simulink model "working_kalman_old"  (R2025b)
settings: Solver=FixedStepDiscrete  StartTime=0.0  StopTime=+inf  FixedStep=simulink_Ts  RelTol=1e-3  EnableMultiTasking=on
InitFcn:
  | InitSensorFusion
values from neighbouring files (symbols this model uses):
  avg_order = 2    [InitSensorFusion_old.m]
  d = 0.15*sqrt(2)/2    [InitSensorFusion_old.m]
  friction_offset = 0.0001    [InitSensorFusion_old.m]
  friction_slope = 0.023e-3    (= 2.3e-05)    [InitSensorFusion_old.m]
  g = 9.81    [InitSensorFusion_old.m]
  Ic0 = Is0 + Iw0 - Iwg    [InitSensorFusion_old.m]
  ICM42_g = 9.8121    [InitSensorFusion_old.m]
  ICM42_gyr_offset = [-0.1319, -0.6878, 0.1737]    [InitSensorFusion_old.m]
  ICM42_params = params_1period    [InitSensorFusion_old.m]
  init_acc_bias = [0 0 0]'    [InitSensorFusion_old.m]
  init_P = P_initial    (= 10)    [InitSensorFusion_old.m]
  init_rot_quat = [0 0 0 1]'    [InitSensorFusion_old.m]
  kalman_Ts = 0.01    [InitSensorFusion_old.m]
  KV = 330    [InitSensorFusion_old.m]
  mc = mw + ms    (= 0.55)    [InitSensorFusion_old.m]
  sensor_Ts = 0.01    [InitSensorFusion_old.m]
  simulink_Ts = 0.01    [InitSensorFusion_old.m]
  stateInit = StateEnum.Initialization    [InitSensorFusion_old.m]
undefined symbols (not defined in the file or in its folder): init_time, StateEnum
libraries: mbedblockslib x24, stmnucleof7lib x5, nucleoutilitieslib x5, canmsglib x4, simulink x3, visionstatistics x2
(part 1 of 2)
settings Model: SimulationMode=external  ExtModeTrigDuration=10  Creator=dozav  LastModifiedBy=dozav
settings SolverCC: AutoInsertRateTranBlk=on
settings DataIOCC: SaveOutput=off  DSMLogging=off  ReturnWorkspaceOutputs=off  LoggingFileName=loggedData.mat
settings OptimizationCC: DefaultParameterBehavior=Inlined  EnhancedBackFolding=on  PassReuseOutputArgsAs=Individual arguments  ZeroExternalMemoryAtStartup=off  ZeroInternalMemoryAtStartup=off  MaxStackSize=64  OptimizeBlockOrder=speed  DifferentSizesBufferReuse=on  OptimizationCustomize=off  EfficientTunableParamExpr=on
settings DebuggingCC: ParameterTunabilityLossMsg=error
settings HardwareCC: ProdBitPerPointer=32.0  ProdBitPerSizeT=32.0  ProdBitPerPtrDiffT=32.0  ProdLargestAtomicInteger=Long  ProdLargestAtomicFloat=Double  ProdWordSize=32.0  ProdLongLongMode=on  ProdHWDeviceType=ARM Compatible->ARM Cortex-M
settings ModelReferenceCC: UpdateModelReferenceTargets=Force
settings SFSimCC: MATLABDynamicMemAlloc=off
settings RTWCC: SystemTargetFile=ert.tlc  HardwareBoard=STM32 Nucleo F767ZI  TemplateMakefile=ert_default_tmf  Toolchain=GNU Tools for ARM Embedded Processors  Description=Embedded Coder
settings CodeAppCC: ForceParamTrailComments=on  IgnoreCustomStorageClasses=off  OperatorAnnotations=on  SimulinkDataObjDesc=on  SFDataObjDesc=on  InsertBlockDesc=on
settings ERTTargetCC: ExtModeTransport=3.0  ExtModeStaticAlloc=on  ExtModeStaticAllocSize=2000.0  ExtModeMexFile=ext_xcp  ExtModeIntrfLevel=Level2 - Open  TargetLangStandard=C99 (ISO)

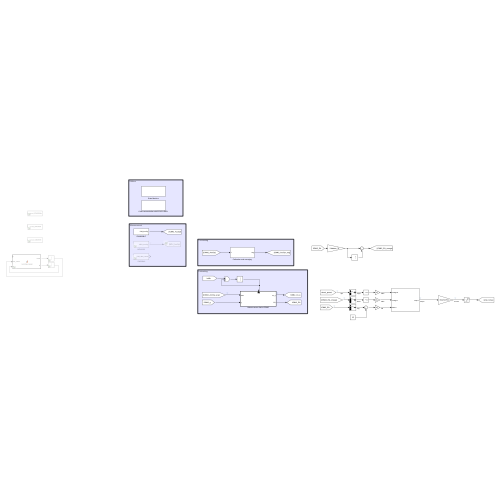
[thumbnail: Simulink's stored preview of the top-level diagram]
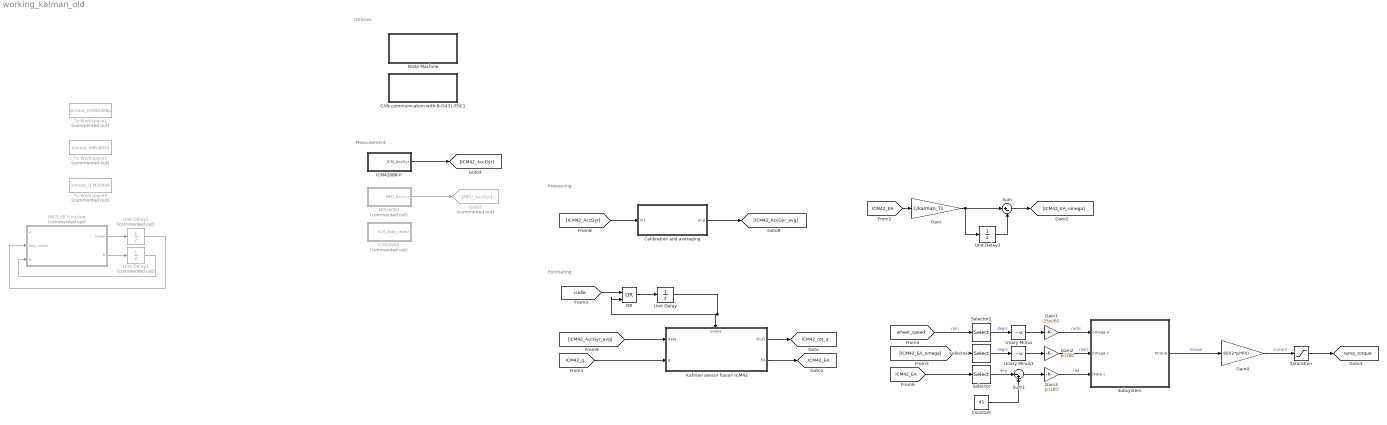
== system working_kalman_old ==
  note: Utilities
  note: Estimating
  note: Processing
  note: Measurement
  CAN communication with B-G431-ESC1 : Subsystem
  Calibration and averaging : Subsystem
  Constant : Constant  Value=45
  Gain : Gain  Gain=1/kalman_Ts
  Gain1 : Gain  Gain=2*pi/60
  Gain2 : Gain  Gain=pi/180
  Gain3 : Gain  Gain=pi/180
  Gain4 : Gain  Gain=60/(2*pi*KV)
  Goto5 : Goto  Commented=on  GotoTag=MPU_AccGyr
  ICM20948 : Subsystem  Commented=on
  ICM42688-P : Subsystem
  Kalman sensor fusion ICM42 : Subsystem
  MATLAB Function : MATLAB Function  Commented=on  TreatAsAtomicUnit=on
  MPU6050 : Subsystem  Commented=on
  OR : Logic  Operator=OR  IconShape=distinctive  AllPortsSameDT=off  OutDataTypeStr=boolean
  Saturation : Saturate  UpperLimit=1.5  LowerLimit=-1.5
  Selector : Selector  InputPortWidth=3  IndexOptions=Index vector (dialog)  Indices=[1]  OutputSizes=1
  Selector1 : Selector  InputPortWidth=3  IndexOptions=Index vector (dialog)  Indices=[1]  OutputSizes=1
  Selector2 : Selector  InputPortWidth=2  IndexOptions=Index vector (dialog)  Indices=[1]  OutputSizes=1
  State Machine : Subsystem
  Subsystem : Subsystem
  Sum : Sum  Inputs=|+-
  Sum1 : Sum  Inputs=|-+
  To Workspace1 : ToWorkspace  Commented=on  VariableName=simout_ICM42688p  SampleTime=-1
  To Workspace2 : ToWorkspace  Commented=on  VariableName=simout_MPU6050  SampleTime=-1
  To Workspace3 : ToWorkspace  Commented=on  VariableName=simout_ICM20948  SampleTime=-1
  Unary Minus : UnaryMinus
  Unary Minus1 : UnaryMinus
  Unit Delay : UnitDelay  SampleTime=-1  HasFrameUpgradeWarning=on
  Unit Delay1 : UnitDelay  Commented=on  SampleTime=-1  HasFrameUpgradeWarning=on
  Unit Delay2 : UnitDelay  Commented=on  SampleTime=-1  HasFrameUpgradeWarning=on
  Unit Delay3 : UnitDelay  InitialCondition=zeros(1,3)  SampleTime=kalman_Ts  HasFrameUpgradeWarning=on
  tag scope: ICM42_EA=global, ICM42_rot_q=global, ramp_torque=global
  wires:
  ICM42688-P/1(ICM_AccGyr) -> [ICM42_AccGyr]
  MATLAB Function/2(N) -> Unit Delay1/1
  MATLAB Function/1(mean) -> Unit Delay2/1
  Unit Delay1/1 -> MATLAB Function/3("N ")
  Unit Delay2/1 -> MATLAB Function/2(last_mean)
  [ICM42_g] -> Kalman sensor fusion ICM42/2(g)
  [ICM42_AccGyr_avg] -> Kalman sensor fusion ICM42/1(data)
  MPU6050/1(MPU_AccGyr) -> Goto5/1
  [isIdle] -> OR/1
  OR/1 -> Unit Delay/1
  Unit Delay/1 -> OR/2, Kalman sensor fusion ICM42/Enable
  [ICM42_AccGyr] -> Calibration and averaging/1(In1)
  Calibration and averaging/1(avg) -> [ICM42_AccGyr_avg]
  Kalman sensor fusion ICM42/1(Out1) -> [ICM42_rot_q]
  Kalman sensor fusion ICM42/2(EA) -> [ICM42_EA]
  [ICM42_EA] -> Gain/1
  Unit Delay3/1 -> Sum/2
  Sum/1 -> [ICM42_EA_omega]
  Gain/1 -> Sum/1, Unit Delay3/1
  [ICM42_EA] -> Selector/1
  [ICM42_EA_omega] -> Selector1/1
  [wheel_speed] -> Selector2/1  "rpm"
  Selector1/1 -> Unary Minus1/1  "deg/s"
  Gain1/1 -> Subsystem/1(omega w)  "rad/s"
  Gain2/1 -> Subsystem/2(omega c)  "rad/s"
  Gain3/1 -> Subsystem/3(theta c)  "rad"
  Selector2/1 -> Unary Minus/1  "deg/s"
  Subsystem/1(torque) -> Gain4/1  "torque"
  Gain4/1 -> Saturation/1  "current"
  Saturation/1 -> [ramp_torque]
  Unary Minus/1 -> Gain1/1
  Unary Minus1/1 -> Gain2/1
  Selector/1 -> Sum1/1  "deg"
  Sum1/1 -> Gain3/1
  Constant/1 -> Sum1/2

== system working_kalman_old/CAN communication with B-G431-ESC1 ==
  Receive CAN Messages : Subsystem
  Send CAN Messages : Subsystem

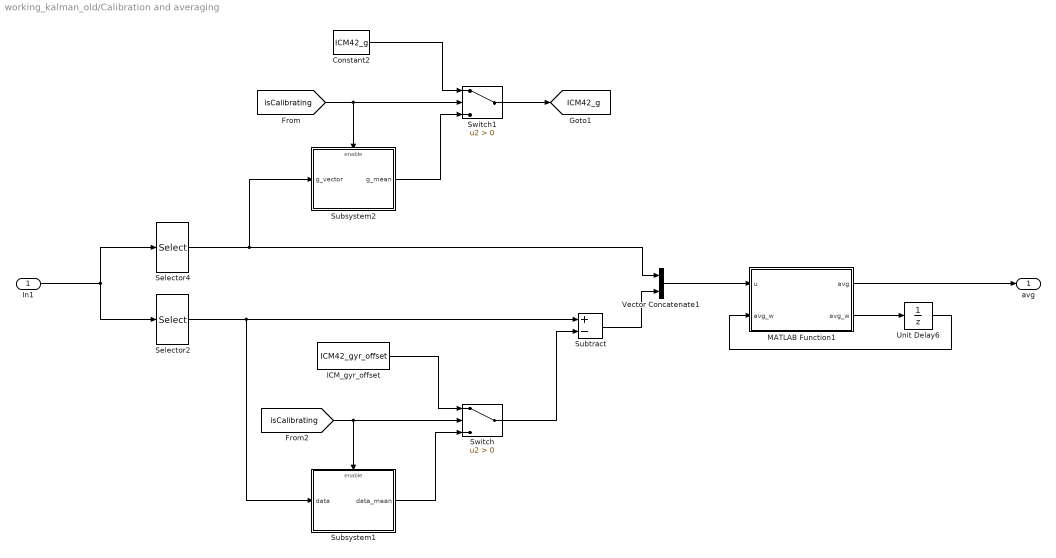
== system working_kalman_old/Calibration and averaging ==
  In1 : Inport
  Constant2 : Constant  Value=ICM42_g  SampleTime=-1
  ICM_gyr_offset : Constant  Value=ICM42_gyr_offset  SampleTime=-1
  MATLAB Function1 : MATLAB Function  TreatAsAtomicUnit=on
  Selector2 : Selector  InputPortWidth=6  IndexOptions=Starting index (dialog)  Indices=[4]  OutputSizes=3
  Selector4 : Selector  InputPortWidth=6  IndexOptions=Starting index (dialog)  Indices=[1]  OutputSizes=3
  Subsystem1 : Subsystem
  Subsystem2 : Subsystem
  Subtract : Sum  Inputs=+-
  Switch : Switch  Criteria=u2 > Threshold  SaturateOnIntegerOverflow=off  InputSameDT=off
  Switch1 : Switch  Criteria=u2 > Threshold  SaturateOnIntegerOverflow=off  InputSameDT=off
  Unit Delay6 : UnitDelay  InitialCondition=zeros(avg_order, 6)  SampleTime=-1  HasFrameUpgradeWarning=on
  Vector Concatenate1 : Concatenate
  avg : Outport
  tag scope: ICM42_g=global
  wires:
  Switch/1 -> Subtract/2
  MATLAB Function1/1(avg) -> avg/1
  Constant2/1 -> Switch1/1
  Subsystem1/1(data_mean) -> Switch/3
  Selector4/1 -> Vector Concatenate1/1, Subsystem2/1(g_vector)
  In1/1 -> Selector2/1, Selector4/1
  MATLAB Function1/2(avg_w) -> Unit Delay6/1
  Subtract/1 -> Vector Concatenate1/2
  Vector Concatenate1/1 -> MATLAB Function1/1(u)
  Switch1/1 -> [ICM42_g]
  Selector2/1 -> Subtract/1, Subsystem1/1(data)
  [isCalibrating] -> Subsystem2/Enable, Switch1/2
  Subsystem2/1(g_mean) -> Switch1/3
  Unit Delay6/1 -> MATLAB Function1/2("avg_w ")
  ICM_gyr_offset/1 -> Switch/1
  [isCalibrating] -> Switch/2, Subsystem1/Enable

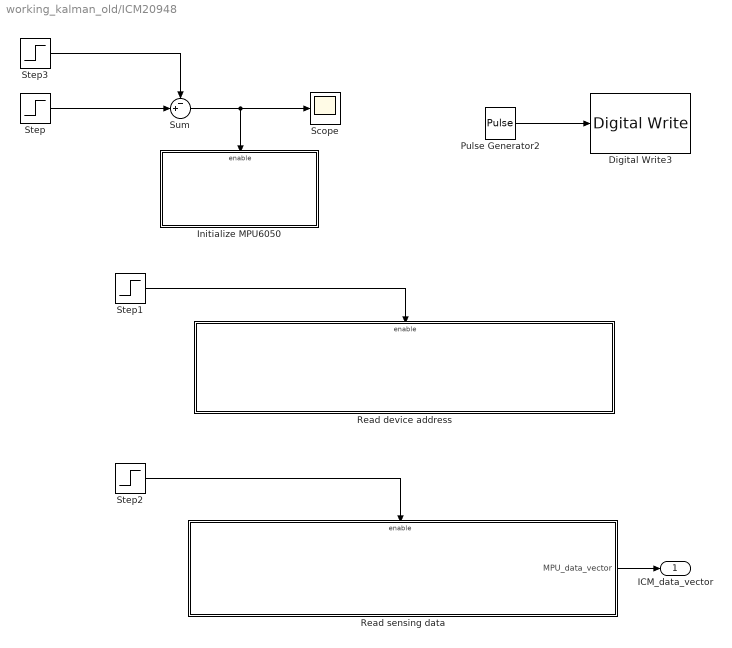
== system working_kalman_old/ICM20948 ==
  Digital Write3 : mbedblockslib/Digital Write  Pin=LED3  Direction=output
      settings: LibrarySourceBlock=stmnucleorootlib/Common/Digital Write
  Initialize MPU6050 : Subsystem
  Pulse Generator2 : DiscretePulseGenerator  PulseType=Time based  PulseWidth=50
  Read device address : Subsystem
  Read sensing data : Subsystem
  Scope : Scope
      settings: DataLoggingVariableName=ScopeData5
  Step : Step
  Step1 : Step  Time=2
  Step2 : Step  Time=2
  Step3 : Step  Time=1.5
  Sum : Sum  Inputs=-+|
  ICM_data_vector : Outport
  wires:
  Step2/1 -> Read sensing data/Enable
  Read sensing data/1(MPU_data_vector) -> ICM_data_vector/1
  Sum/1 -> Scope/1, Initialize MPU6050/Enable
  Step/1 -> Sum/2
  Step1/1 -> Read device address/Enable
  Step3/1 -> Sum/1
  Pulse Generator2/1 -> Digital Write3/1

== system working_kalman_old/ICM42688-P ==
  Measurement : Subsystem
  OR : Logic  Operator=OR  IconShape=distinctive  AllPortsSameDT=off  OutDataTypeStr=boolean
  Range and sensitivity : Subsystem  Priority=1
  Selector : Selector  InputPortWidth=7  IndexOptions=Starting index (dialog)  Indices=[2]  OutputSizes=6
  Step1 : Step  Time=init_time - 3
  Step3 : Step  Time=init_time - 4
  Unit Delay : UnitDelay  SampleTime=-1  HasFrameUpgradeWarning=on
  Waking up : Subsystem  Priority=2
  ICM_AccGyr : Outport
  wires:
  Step1/1 -> Waking up/Trigger
  Step3/1 -> Range and sensitivity/Trigger
  OR/1 -> Unit Delay/1
  Unit Delay/1 -> OR/2, Measurement/Enable
  Measurement/1(ICM_data_vector) -> Selector/1
  [isCalibrating] -> OR/1
  Selector/1 -> ICM_AccGyr/1

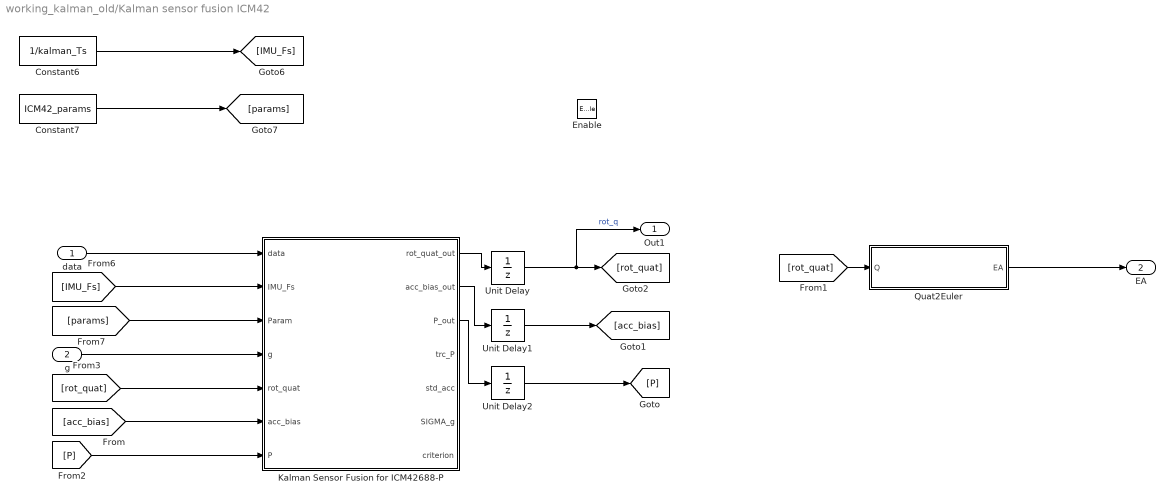
== system working_kalman_old/Kalman sensor fusion ICM42 ==
  data : Inport
  g : Inport  Port=2
  Enable : EnablePort
  Constant6 : Constant  Value=1/kalman_Ts  SampleTime=-1
  Constant7 : Constant  Value=ICM42_params  SampleTime=-1
  Kalman Sensor Fusion for ICM42688-P : MATLAB Function  TreatAsAtomicUnit=on
  Quat2Euler : MATLAB Function  TreatAsAtomicUnit=on
  Unit Delay : UnitDelay  InitialCondition=init_rot_quat  SampleTime=-1  HasFrameUpgradeWarning=on
  Unit Delay1 : UnitDelay  InitialCondition=init_acc_bias  SampleTime=-1  HasFrameUpgradeWarning=on
  Unit Delay2 : UnitDelay  InitialCondition=init_P*eye(7)  SampleTime=-1  HasFrameUpgradeWarning=on
  Out1 : Outport
  EA : Outport  Port=2
  wires:
  [acc_bias] -> Kalman Sensor Fusion for ICM42688-P/6(acc_bias)
  [P] -> Kalman Sensor Fusion for ICM42688-P/7(P)
  Unit Delay/1 -> Out1/1, [rot_quat]  "rot_q"
  [IMU_Fs] -> Kalman Sensor Fusion for ICM42688-P/2(IMU_Fs)
  Kalman Sensor Fusion for ICM42688-P/1(rot_quat_out) -> Unit Delay/1
  [rot_quat] -> Kalman Sensor Fusion for ICM42688-P/5(rot_quat)
  Kalman Sensor Fusion for ICM42688-P/2(acc_bias_out) -> Unit Delay1/1
  Kalman Sensor Fusion for ICM42688-P/3(P_out) -> Unit Delay2/1
  [params] -> Kalman Sensor Fusion for ICM42688-P/3(Param)
  Constant6/1 -> [IMU_Fs]
  Unit Delay1/1 -> [acc_bias]
  Unit Delay2/1 -> [P]
  Constant7/1 -> [params]
  data/1 -> Kalman Sensor Fusion for ICM42688-P/1(data)
  [rot_quat] -> Quat2Euler/1(Q)
  g/1 -> Kalman Sensor Fusion for ICM42688-P/4(g)
  Quat2Euler/1(EA) -> EA/1

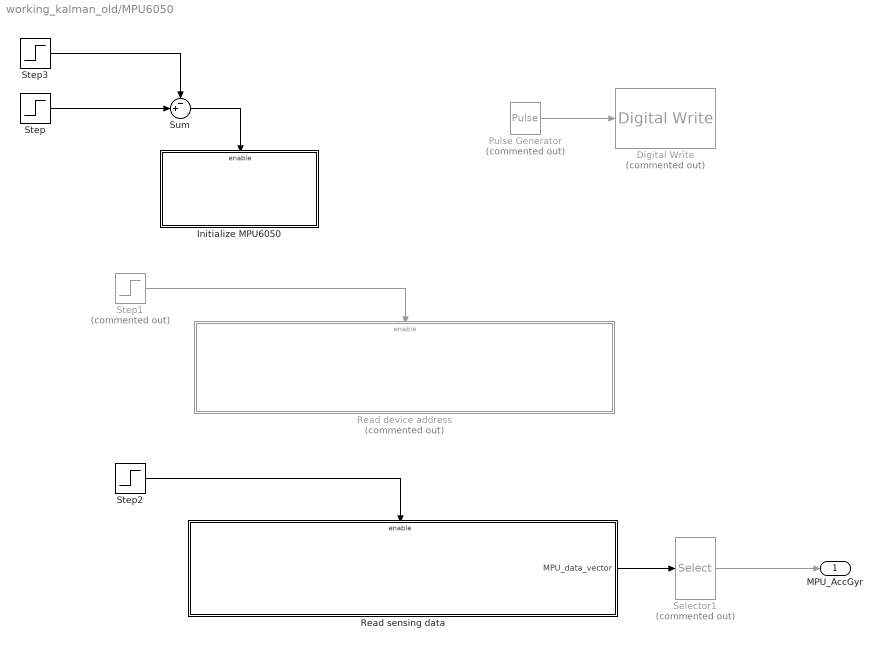
== system working_kalman_old/MPU6050 ==
  Digital Write : mbedblockslib/Digital Write  Commented=on  Pin=LED1  Direction=output
      settings: LibrarySourceBlock=stmnucleorootlib/Common/Digital Write
  Initialize MPU6050 : Subsystem
  Pulse Generator : DiscretePulseGenerator  Commented=on  PulseType=Time based  Period=0.5  PulseWidth=50
  Read device address : Subsystem  Commented=on
  Read sensing data : Subsystem
  Selector1 : Selector  Commented=on  InputPortWidth=7  IndexOptions=Index vector (dialog)  Indices=[1 2 3 5 6 7]  OutputSizes=6
  Step : Step
  Step1 : Step  Commented=on  Time=2
  Step2 : Step  Time=2
  Step3 : Step  Time=1.5
  Sum : Sum  Inputs=-+|
  MPU_AccGyr : Outport
  wires:
  Step2/1 -> Read sensing data/Enable
  Read sensing data/1(MPU_data_vector) -> Selector1/1
  Sum/1 -> Initialize MPU6050/Enable
  Step/1 -> Sum/2
  Pulse Generator/1 -> Digital Write/1
  Step1/1 -> Read device address/Enable
  Step3/1 -> Sum/1
  Selector1/1 -> MPU_AccGyr/1

== system working_kalman_old/State Machine ==
  State Recognition : Subsystem
  State Signalizition : Subsystem
  State Updates : Subsystem

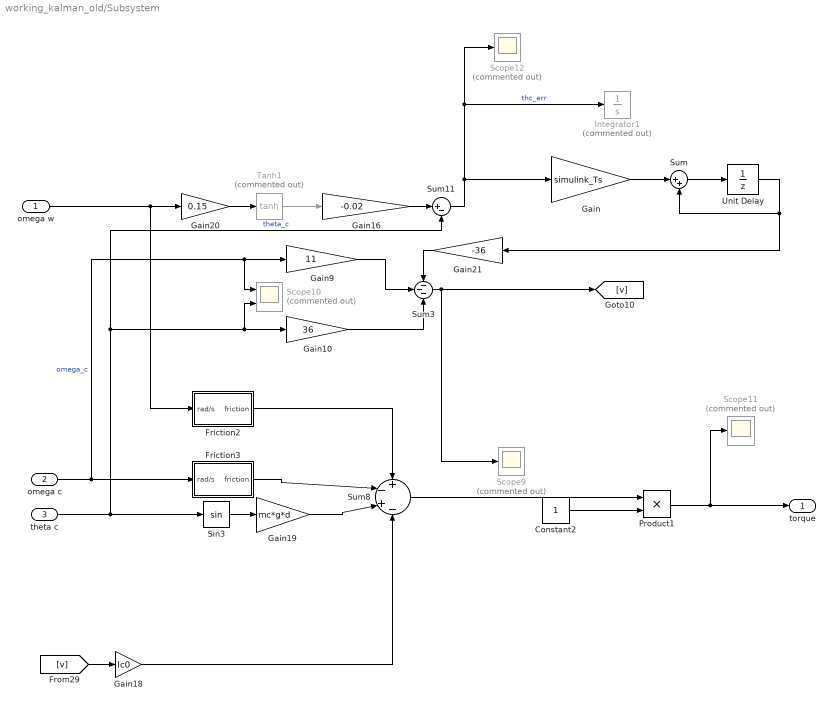
== system working_kalman_old/Subsystem ==
  omega w : Inport
  omega c : Inport  Port=2
  theta c : Inport  Port=3
  Constant2 : Constant
  Friction2 : Subsystem
  Friction3 : Subsystem
  Gain : Gain  Gain=simulink_Ts
  Gain10 : Gain  Gain=36
  Gain16 : Gain  Gain=-0.02
  Gain18 : Gain  Gain=Ic0
  Gain19 : Gain  Gain=mc*g*d
  Gain20 : Gain  Gain=0.15
  Gain21 : Gain  Gain=-36
  Gain9 : Gain  Gain=11
  Integrator1 : Integrator  Commented=on
  Product1 : Product
  Scope10 : Scope  Commented=on  NumInputPorts=2
      settings: ActiveDisplayYMinimum=-0.04851  ActiveDisplayYMaximum=0.02163
  Scope11 : Scope  Commented=on
      settings: ActiveDisplayYMinimum=-0.30129  ActiveDisplayYMaximum=1.03269  DataLoggingVariableName=ScopeData2
  Scope12 : Scope  Commented=on
      settings: ActiveDisplayYMinimum=-0.23331  ActiveDisplayYMaximum=0.0687  DataLoggingVariableName=ScopeData3
  Scope9 : Scope  Commented=on
      settings: ActiveDisplayYMinimum=-0.82358  ActiveDisplayYMaximum=0.21225  DataLoggingVariableName=ScopeData4
  Sin3 : Trigonometry
  Sum : Sum  Inputs=|++
  Sum11 : Sum  Inputs=|+-
  Sum3 : Sum  Inputs=---
  Sum8 : Sum  Inputs=+|-|+|-
  Tanh1 : Trigonometry  Commented=on  Operator=tanh
  Unit Delay : UnitDelay  SampleTime=-1  HasFrameUpgradeWarning=on
  torque : Outport
  wires:
  omega c/1 -> Scope10/1, Gain9/1, Friction3/1(rad/s)  "omega_c"
  Sin3/1 -> Gain19/1
  Gain19/1 -> Sum8/3
  Sum3/1 -> Scope9/1, [v]
  Friction2/1(friction) -> Sum8/1
  Product1/1 -> torque/1, Scope11/1
  Gain18/1 -> Sum8/4
  Gain16/1 -> Sum11/1
  Gain10/1 -> Sum3/3
  Constant2/1 -> Product1/2
  Sum11/1 -> Gain/1, Scope12/1, Integrator1/1  "thc_err"
  Tanh1/1 -> Gain16/1
  Friction3/1(friction) -> Sum8/2
  Gain21/1 -> Sum3/1
  Gain20/1 -> Tanh1/1
  [v] -> Gain18/1
  omega w/1 -> Friction2/1(rad/s), Gain20/1
  Sum8/1 -> Product1/1
  theta c/1 -> Scope10/2, Gain10/1, Sum11/2, Sin3/1  "theta_c"
  Gain9/1 -> Sum3/2
  Sum/1 -> Unit Delay/1
  Gain/1 -> Sum/1
  Unit Delay/1 -> Sum/2, Gain21/1

== system working_kalman_old/CAN communication with B-G431-ESC1/Receive CAN Messages ==
  CAN Receive : stmnucleof7lib/CAN Receive  CANModule=1  OutputType=Unpacked  ReadSource=FIFO 0  SampleTime=kalman_Ts  OutputIdType=off  RemoteFrame=off  OutputStatus=off
  Compare To Constant1 : simulink/Logic and Bit Operations/Compare To Constant  relop===  const=hex2dec('104')  OutDataTypeStr=boolean
  Subsystem3 : Subsystem
  tag scope: wheel_speed=global
  wires:
  [CAN_data] -> Subsystem3/1(In1)
  CAN Receive/3 -> [CAN_data]
  CAN Receive/1 -> [CAN_id]
  [CAN_id] -> Compare To Constant1/1
  Compare To Constant1/1 -> Subsystem3/Enable
  Subsystem3/1(Out1) -> [wheel_speed]

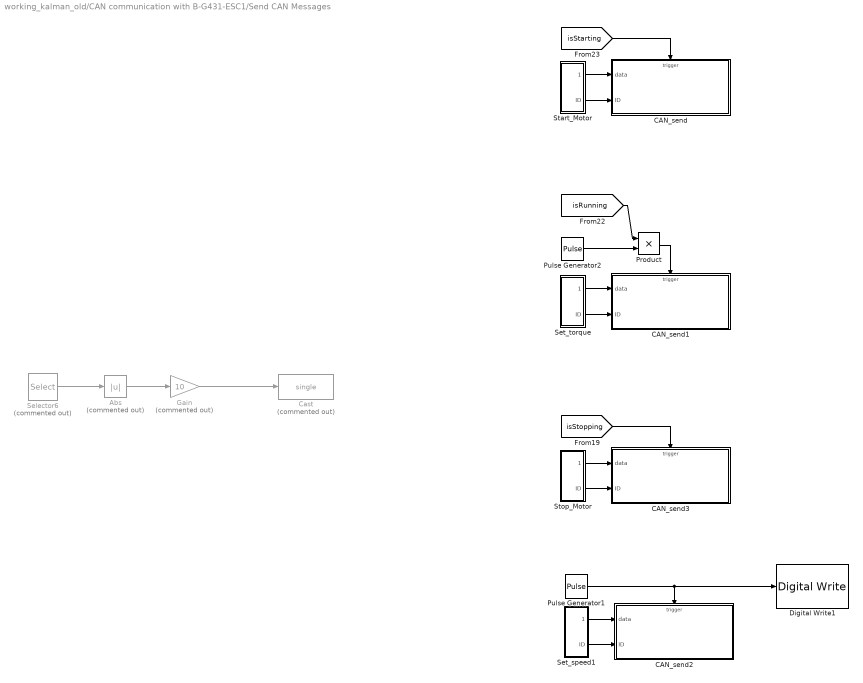
== system working_kalman_old/CAN communication with B-G431-ESC1/Send CAN Messages ==
  Abs : Abs  Commented=on  SaturateOnIntegerOverflow=off
  CAN_send : Subsystem
  CAN_send1 : Subsystem
  CAN_send2 : Subsystem
  CAN_send3 : Subsystem
  Cast : DataTypeConversion  Commented=on  OutDataTypeStr=single  SaturateOnIntegerOverflow=off  RndMeth=Floor
  Digital Write1 : mbedblockslib/Digital Write  Pin=LED1  Direction=output
      settings: LibrarySourceBlock=stmnucleorootlib/Common/Digital Write
  Gain : Gain  Commented=on  Gain=10
  Product : Product
  Pulse Generator1 : DiscretePulseGenerator  PulseType=Time based  Period=0.1  PulseWidth=50
  Pulse Generator2 : DiscretePulseGenerator  PulseType=Time based  Period=2*simulink_Ts  PulseWidth=50
  Selector6 : Selector  Commented=on  InputPortWidth=3  IndexOptions=Index vector (dialog)  Indices=[1]  OutputSizes=1
  Set_speed1 : Subsystem
  Set_torque : Subsystem
  Start_Motor : Subsystem
  Stop_Motor : Subsystem
  wires:
  Set_torque/2(ID) -> CAN_send1/2(ID)
  Selector6/1 -> Abs/1
  Set_speed1/1(data) -> CAN_send2/1(data)
  Stop_Motor/1(data) -> CAN_send3/1(data)
  Set_torque/1(data) -> CAN_send1/1(data)
  [isStopping] -> CAN_send3/Trigger
  Pulse Generator1/1 -> Digital Write1/1, CAN_send2/Trigger
  Start_Motor/2(ID) -> CAN_send/2(ID)
  [isStarting] -> CAN_send/Trigger
  [isRunning] -> Product/1
  Gain/1 -> Cast/1
  Start_Motor/1(data) -> CAN_send/1(data)
  Pulse Generator2/1 -> Product/2
  Abs/1 -> Gain/1
  Product/1 -> CAN_send1/Trigger
  Stop_Motor/2(ID) -> CAN_send3/2(ID)
  Set_speed1/2(ID) -> CAN_send2/2(ID)

== system working_kalman_old/Calibration and averaging/Subsystem1 ==
  data : Inport
  Enable : EnablePort
  2-D Mean3 : visionstatistics/2-D Mean  run=on  reset_popup=Rising edge  directionMode=Each row  dimension=1  treatSBRowAsCol=on  outputLastDataTypeStr=Inherit: Same as accumulator  accumMode=Binary point scaling  accumWordLength=32  accumFracLength=0  accumLastDataTypeStr=fixdt([],32,0)  roiEnable=off  roiType=Rectangles  roiPortion=Entire ROI  roiOutput=Individual statistics for each ROI  roiFlag=off  roundingMode=Floor  overflowMode=off  accumDataTypeStr=fixdt([],32,0)  outputDataTypeStr=Inherit: Same as accumulator  outputMin=[]  outputMax=[]
  Cast To Boolean : DataTypeConversion  OutDataTypeStr=boolean  SaturateOnIntegerOverflow=off  RndMeth=Floor
  Sum of Elements : Sum  Inputs=+
  data_mean : Outport
  wires:
  2-D Mean3/1 -> data_mean/1
  data/1 -> 2-D Mean3/1, Sum of Elements/1
  Sum of Elements/1 -> Cast To Boolean/1
  Cast To Boolean/1 -> 2-D Mean3/2

== system working_kalman_old/Calibration and averaging/Subsystem2 ==
  g_vector : Inport
  Enable : EnablePort
  2-D Mean3 : visionstatistics/2-D Mean  run=on  reset_popup=Rising edge  directionMode=Each row  dimension=1  treatSBRowAsCol=on  outputLastDataTypeStr=Inherit: Same as accumulator  accumMode=Binary point scaling  accumWordLength=32  accumFracLength=0  accumLastDataTypeStr=fixdt([],32,0)  roiEnable=off  roiType=Rectangles  roiPortion=Entire ROI  roiOutput=Individual statistics for each ROI  roiFlag=off  roundingMode=Floor  overflowMode=off  accumDataTypeStr=fixdt([],32,0)  outputDataTypeStr=Inherit: Same as accumulator  outputMin=[]  outputMax=[]
  Cast To Boolean : DataTypeConversion  OutDataTypeStr=boolean  SaturateOnIntegerOverflow=off  RndMeth=Floor
  MATLAB Function1 : MATLAB Function  TreatAsAtomicUnit=on
  Sum of Elements : Sum  Inputs=+
  g_mean : Outport
  wires:
  2-D Mean3/1 -> g_mean/1
  g_vector/1 -> Sum of Elements/1, MATLAB Function1/1(g_vector)
  MATLAB Function1/1(g_scalar) -> 2-D Mean3/1
  Sum of Elements/1 -> Cast To Boolean/1
  Cast To Boolean/1 -> 2-D Mean3/2

== system working_kalman_old/ICM20948/Initialize MPU6050 ==
  Enable : EnablePort
  Accelerometer scale : mbedblockslib/I2C Controller Write  Commented=on  I2CModule=0  Mode=Master  SlaveAddress=hex2dec('68')  SlaveByteOrder=BigEndian  Direction=Transmitter  RegisterAddressMode=on  RegisterAddress=hex2dec('1C')  SlaveDataType=uint8  DataLength=2  NoAck=off  RepeatedStart=off  OutputStatus=on
      settings: LibrarySourceBlock=stmnucleorootlib/Common/I2C Controller Write
  Constant : Constant  Commented=on  Value=0b00000000
  Constant1 : Constant  Commented=on  Value=0b00001000
  Constant2 : Constant  Commented=on  Value=0b00010000
  Display1 : Display  Commented=on
  Display2 : Display  Commented=on
  Display5 : Display  Commented=on
  Gyroscope scale : mbedblockslib/I2C Controller Write  Commented=on  I2CModule=0  Mode=Master  SlaveAddress=hex2dec('68')  SlaveByteOrder=BigEndian  Direction=Transmitter  RegisterAddressMode=on  RegisterAddress=hex2dec('1B')  SlaveDataType=uint8  DataLength=2  NoAck=off  RepeatedStart=off  OutputStatus=on
      settings: LibrarySourceBlock=stmnucleorootlib/Common/I2C Controller Write
  Wake up : mbedblockslib/I2C Controller Write  Commented=on  I2CModule=0  Mode=Master  SlaveAddress=hex2dec('68')  SlaveByteOrder=BigEndian  Direction=Transmitter  RegisterAddressMode=on  RegisterAddress=hex2dec('6B')  SlaveDataType=uint8  DataLength=2  NoAck=off  RepeatedStart=off  OutputStatus=on
      settings: LibrarySourceBlock=stmnucleorootlib/Common/I2C Controller Write
  wires:
  Constant/1 -> Wake up/1
  Wake up/1 -> Display5/1
  Gyroscope scale/1 -> Display1/1
  Constant1/1 -> Gyroscope scale/1
  Constant2/1 -> Accelerometer scale/1
  Accelerometer scale/1 -> Display2/1

== system working_kalman_old/ICM20948/Read device address ==
  Enable : EnablePort
  Display1 : Display  Commented=on
  Display2 : Display
  Display3 : Display  Commented=on
  Scope1 : Scope  Commented=on
      settings: DataLoggingVariableName=ScopeData6
  Scope2 : Scope  Commented=on
      settings: DataLoggingVariableName=ScopeData7
  Scope3 : Scope
      settings: DataLoggingVariableName=ScopeData2
  WHO_AM_I_0x69 : mbedblockslib/I2C Controller Read  I2CModule=2  Mode=Master  SlaveAddress=hex2dec('69')  SlaveByteOrder=BigEndian  Direction=Receiver  RegisterAddressMode=on  RegisterAddress=hex2dec('0')  SlaveDataType=uint8  DataLength=1  NoAck=off  RepeatedStart=off  OutputStatus=on  SampleTime=0.1
      settings: LibrarySourceBlock=stmnucleorootlib/Common/I2C Controller Read
  acc_scale : mbedblockslib/I2C Controller Read  Commented=on  I2CModule=0  Mode=Master  SlaveAddress=hex2dec('68')  SlaveByteOrder=BigEndian  Direction=Receiver  RegisterAddressMode=on  RegisterAddress=hex2dec('1C')  SlaveDataType=int8  DataLength=1  NoAck=off  RepeatedStart=off  OutputStatus=on  SampleTime=20
      settings: LibrarySourceBlock=stmnucleorootlib/Common/I2C Controller Read
  gyr_scale : mbedblockslib/I2C Controller Read  Commented=on  I2CModule=0  Mode=Master  SlaveAddress=hex2dec('68')  SlaveByteOrder=BigEndian  Direction=Receiver  RegisterAddressMode=on  RegisterAddress=hex2dec('1B')  SlaveDataType=int8  DataLength=1  NoAck=off  RepeatedStart=off  OutputStatus=on  SampleTime=20
      settings: LibrarySourceBlock=stmnucleorootlib/Common/I2C Controller Read
  wires:
  WHO_AM_I_0x69/2 -> Display2/1
  WHO_AM_I_0x69/1 -> Scope3/1
  gyr_scale/1 -> Scope1/1
  gyr_scale/2 -> Display1/1
  acc_scale/1 -> Scope2/1
  acc_scale/2 -> Display3/1

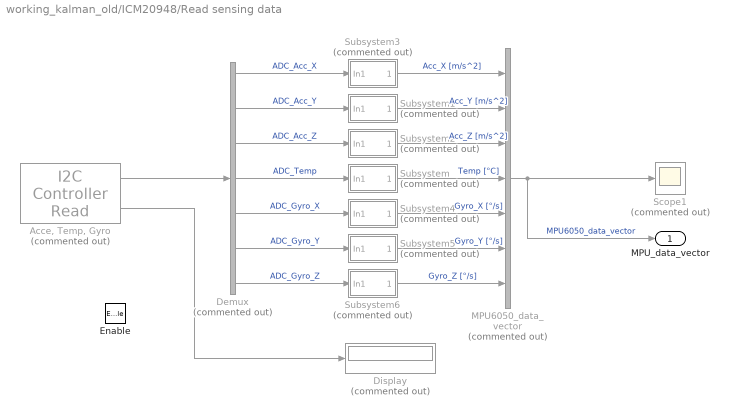
== system working_kalman_old/ICM20948/Read sensing data ==
  Enable : EnablePort
  "Acce, Temp, Gyro" : mbedblockslib/I2C Controller Read  Commented=on  I2CModule=0  Mode=Master  SlaveAddress=hex2dec('68')  SlaveByteOrder=BigEndian  Direction=Receiver  RegisterAddressMode=on  RegisterAddress=hex2dec('3B')  SlaveDataType=int16  DataLength=7  NoAck=off  RepeatedStart=off  OutputStatus=on  SampleTime=0.1
      settings: LibrarySourceBlock=stmnucleorootlib/Common/I2C Controller Read
  Demux : Demux  Commented=on  Outputs=7
  Display : Display  Commented=on
  MPU6050_data_vector : Mux  Commented=on  Inputs=7
  Scope1 : Scope  Commented=on
  Subsystem : Subsystem  Commented=on
  Subsystem1 : Subsystem  Commented=on
  Subsystem2 : Subsystem  Commented=on
  Subsystem3 : Subsystem  Commented=on
  Subsystem4 : Subsystem  Commented=on
  Subsystem5 : Subsystem  Commented=on
  Subsystem6 : Subsystem  Commented=on
  MPU_data_vector : Outport
  wires:
  "Acce, Temp, Gyro"/2 -> Display/1
  "Acce, Temp, Gyro"/1 -> Demux/1
  Demux/1 -> Subsystem3/1(In1)  "ADC_Acc_X"
  Demux/2 -> Subsystem1/1(In1)  "ADC_Acc_Y"
  Demux/3 -> Subsystem2/1(In1)  "ADC_Acc_Z"
  Demux/4 -> Subsystem/1(In1)  "ADC_Temp"
  Demux/5 -> Subsystem4/1(In1)  "ADC_Gyro_X"
  Demux/6 -> Subsystem5/1(In1)  "ADC_Gyro_Y"
  Demux/7 -> Subsystem6/1(In1)  "ADC_Gyro_Z"
  Subsystem6/1(Out1) -> MPU6050_data_vector/7  "Gyro_Z [°/s]"
  Subsystem5/1(Out1) -> MPU6050_data_vector/6  "Gyro_Y [°/s]"
  Subsystem4/1(Out1) -> MPU6050_data_vector/5  "Gyro_X [°/s]"
  Subsystem/1(Out1) -> MPU6050_data_vector/4  "Temp [°C]"
  Subsystem2/1(Out1) -> MPU6050_data_vector/3  "Acc_Z [m/s^2]"
  Subsystem1/1(Out1) -> MPU6050_data_vector/2  "Acc_Y [m/s^2]"
  Subsystem3/1(Out1) -> MPU6050_data_vector/1  "Acc_X [m/s^2]"
  MPU6050_data_vector/1 -> Scope1/1, MPU_data_vector/1  "MPU6050_data_vector"

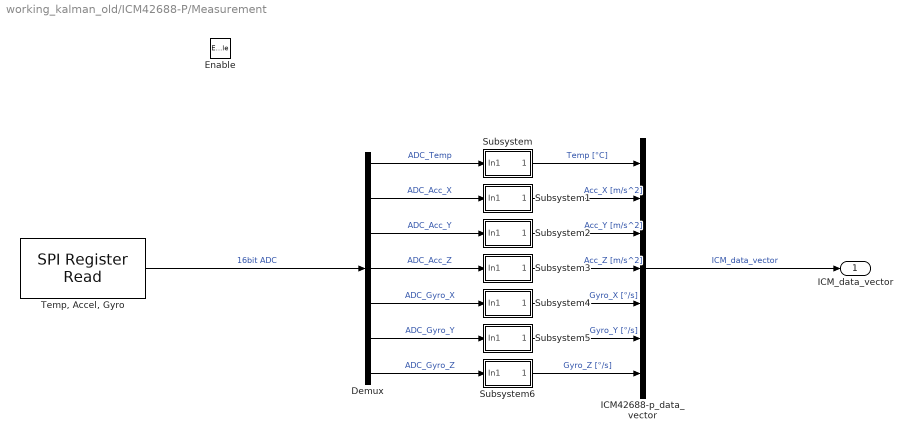
== system working_kalman_old/ICM42688-P/Measurement ==
  Enable : EnablePort
  Demux : Demux  Outputs=7
  ICM42688-p_data_vector : Mux  Inputs=7
  Subsystem : Subsystem
  Subsystem1 : Subsystem
  Subsystem2 : Subsystem
  Subsystem3 : Subsystem
  Subsystem4 : Subsystem
  Subsystem5 : Subsystem
  Subsystem6 : Subsystem
  "Temp, Accel, Gyro" : mbedblockslib/SPI Register Read  Priority=1  SPIModule=0  Mode=Master  BusSpeed=uint32( 1000000 )  Pin=PA_4  FirstBitToTransfer=Most significant bit (MSB)  ClockMode=0  BlockFunction=Read  RegisterAddress=bitor(hex2dec('1D'), hex2dec('80'))  OutputDataType=int16  OutputDataLength=7  SampleTime=sensor_Ts  UseCustomSSPin=Explicit GPIO calls  ActiveLowSSPin=Active low
      settings: LibrarySourceBlock=stmnucleorootlib/Common/SPI Register Read
  ICM_data_vector : Outport
  wires:
  Demux/5 -> Subsystem4/1(In1)  "ADC_Gyro_X"
  Demux/7 -> Subsystem6/1(In1)  "ADC_Gyro_Z"
  Demux/6 -> Subsystem5/1(In1)  "ADC_Gyro_Y"
  Subsystem1/1(Out1) -> ICM42688-p_data_vector/2  "Acc_X [m/s^2]"
  Subsystem3/1(Out1) -> ICM42688-p_data_vector/4  "Acc_Z [m/s^2]"
  Subsystem5/1(Out1) -> ICM42688-p_data_vector/6  "Gyro_Y [°/s]"
  Demux/3 -> Subsystem2/1(In1)  "ADC_Acc_Y"
  Subsystem2/1(Out1) -> ICM42688-p_data_vector/3  "Acc_Y [m/s^2]"
  Subsystem6/1(Out1) -> ICM42688-p_data_vector/7  "Gyro_Z [°/s]"
  Demux/2 -> Subsystem1/1(In1)  "ADC_Acc_X"
  Subsystem4/1(Out1) -> ICM42688-p_data_vector/5  "Gyro_X [°/s]"
  Demux/1 -> Subsystem/1(In1)  "ADC_Temp"
  ICM42688-p_data_vector/1 -> ICM_data_vector/1  "ICM_data_vector"
  Subsystem/1(Out1) -> ICM42688-p_data_vector/1  "Temp [°C]"
  Demux/4 -> Subsystem3/1(In1)  "ADC_Acc_Z"
  "Temp, Accel, Gyro"/1 -> Demux/1  "16bit ADC"

== system working_kalman_old/ICM42688-P/Range and sensitivity ==
  Trigger : TriggerPort  VariantControl=(inherit)  PortDimensions=1
  "ACCEL_FS_SEL and ACCEL_ODR " : mbedblockslib/SPI Register Write  Priority=2  SPIModule=0  Mode=Master  BusSpeed=uint32( 1000000 )  Pin=PA_4  FirstBitToTransfer=Most significant bit (MSB)  ClockMode=0  BlockFunction=Write  RegisterAddress=hex2dec('50')  OutputDataType=int8  OutputDataLength=1  UseCustomSSPin=Explicit GPIO calls  ActiveLowSSPin=Active low
      settings: LibrarySourceBlock=stmnucleorootlib/Common/SPI Register Write
  "BEWARE the reserved bits (1000dps, 1kHz)" : Constant  Value=0b00100110  SampleTime=-1
  "BEWARE the reserved bits (8g, 1kHz)" : Constant  Value=0b00100110  SampleTime=-1
  "GYRO_FS_SEL and GYRO_ODR " : mbedblockslib/SPI Register Write  Priority=1  SPIModule=0  Mode=Master  BusSpeed=uint32( 1000000 )  Pin=PA_4  FirstBitToTransfer=Most significant bit (MSB)  ClockMode=0  BlockFunction=Write  RegisterAddress=hex2dec('4F')  OutputDataType=int8  OutputDataLength=1  UseCustomSSPin=Explicit GPIO calls  ActiveLowSSPin=Active low
      settings: LibrarySourceBlock=stmnucleorootlib/Common/SPI Register Write
  wires:
  "BEWARE the reserved bits (1000dps, 1kHz)"/1 -> "GYRO_FS_SEL and GYRO_ODR "/1
  "BEWARE the reserved bits (8g, 1kHz)"/1 -> "ACCEL_FS_SEL and ACCEL_ODR "/1

== system working_kalman_old/ICM42688-P/Waking up ==
  Trigger : TriggerPort  VariantControl=(inherit)  PortDimensions=1
  BEWARE the reserved bits : Constant  Value=0b00011111  SampleTime=-1
  SPI Register Write : mbedblockslib/SPI Register Write  SPIModule=0  Mode=Master  BusSpeed=uint32( 1000000 )  Pin=PA_4  FirstBitToTransfer=Most significant bit (MSB)  ClockMode=0  BlockFunction=Write  RegisterAddress=hex2dec('4E')  OutputDataType=int8  OutputDataLength=1  UseCustomSSPin=Explicit GPIO calls  ActiveLowSSPin=Active low
      settings: LibrarySourceBlock=stmnucleorootlib/Common/SPI Register Write
  wires:
  BEWARE the reserved bits/1 -> SPI Register Write/1

== system working_kalman_old/MPU6050/Initialize MPU6050 ==
  Enable : EnablePort
  Accelerometer scale : mbedblockslib/I2C Controller Write  I2CModule=0  Mode=Master  SlaveAddress=hex2dec('68')  SlaveByteOrder=BigEndian  Direction=Transmitter  RegisterAddressMode=on  RegisterAddress=hex2dec('1C')  SlaveDataType=uint8  DataLength=2  NoAck=off  RepeatedStart=off  OutputStatus=on
      settings: LibrarySourceBlock=stmnucleorootlib/Common/I2C Controller Write
  Constant : Constant  Value=0b00000000
  Constant1 : Constant  Value=0b00001000
  Constant2 : Constant  Value=0b00010000
  Gyroscope scale : mbedblockslib/I2C Controller Write  I2CModule=0  Mode=Master  SlaveAddress=hex2dec('68')  SlaveByteOrder=BigEndian  Direction=Transmitter  RegisterAddressMode=on  RegisterAddress=hex2dec('1B')  SlaveDataType=uint8  DataLength=2  NoAck=off  RepeatedStart=off  OutputStatus=on
      settings: LibrarySourceBlock=stmnucleorootlib/Common/I2C Controller Write
  Wake up : mbedblockslib/I2C Controller Write  I2CModule=0  Mode=Master  SlaveAddress=hex2dec('68')  SlaveByteOrder=BigEndian  Direction=Transmitter  RegisterAddressMode=on  RegisterAddress=hex2dec('6B')  SlaveDataType=uint8  DataLength=2  NoAck=off  RepeatedStart=off  OutputStatus=on
      settings: LibrarySourceBlock=stmnucleorootlib/Common/I2C Controller Write
  wires:
  Constant/1 -> Wake up/1
  Constant1/1 -> Gyroscope scale/1
  Constant2/1 -> Accelerometer scale/1

== system working_kalman_old/MPU6050/Read device address ==
  Enable : EnablePort
  WHO_AM_I : mbedblockslib/I2C Controller Read  I2CModule=0  Mode=Master  SlaveAddress=hex2dec('68')  SlaveByteOrder=BigEndian  Direction=Receiver  RegisterAddressMode=on  RegisterAddress=hex2dec('75')  SlaveDataType=int8  DataLength=1  NoAck=off  RepeatedStart=off  OutputStatus=on  SampleTime=20
      settings: LibrarySourceBlock=stmnucleorootlib/Common/I2C Controller Read
  acc_scale : mbedblockslib/I2C Controller Read  I2CModule=0  Mode=Master  SlaveAddress=hex2dec('68')  SlaveByteOrder=BigEndian  Direction=Receiver  RegisterAddressMode=on  RegisterAddress=hex2dec('1C')  SlaveDataType=int8  DataLength=1  NoAck=off  RepeatedStart=off  OutputStatus=on  SampleTime=20
      settings: LibrarySourceBlock=stmnucleorootlib/Common/I2C Controller Read
  gyr_scale : mbedblockslib/I2C Controller Read  I2CModule=0  Mode=Master  SlaveAddress=hex2dec('68')  SlaveByteOrder=BigEndian  Direction=Receiver  RegisterAddressMode=on  RegisterAddress=hex2dec('1B')  SlaveDataType=int8  DataLength=1  NoAck=off  RepeatedStart=off  OutputStatus=on  SampleTime=20
      settings: LibrarySourceBlock=stmnucleorootlib/Common/I2C Controller Read

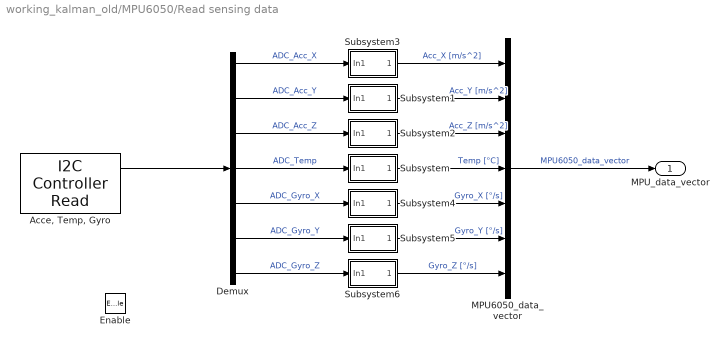
== system working_kalman_old/MPU6050/Read sensing data ==
  Enable : EnablePort
  "Acce, Temp, Gyro" : mbedblockslib/I2C Controller Read  I2CModule=0  Mode=Master  SlaveAddress=hex2dec('68')  SlaveByteOrder=BigEndian  Direction=Receiver  RegisterAddressMode=on  RegisterAddress=hex2dec('3B')  SlaveDataType=int16  DataLength=7  NoAck=off  RepeatedStart=off  OutputStatus=on  SampleTime=sensor_Ts
      settings: LibrarySourceBlock=stmnucleorootlib/Common/I2C Controller Read
  Demux : Demux  Outputs=7
  MPU6050_data_vector : Mux  Inputs=7
  Subsystem : Subsystem
  Subsystem1 : Subsystem
  Subsystem2 : Subsystem
  Subsystem3 : Subsystem
  Subsystem4 : Subsystem
  Subsystem5 : Subsystem
  Subsystem6 : Subsystem
  MPU_data_vector : Outport
  wires:
  "Acce, Temp, Gyro"/1 -> Demux/1
  Demux/1 -> Subsystem3/1(In1)  "ADC_Acc_X"
  Demux/2 -> Subsystem1/1(In1)  "ADC_Acc_Y"
  Demux/3 -> Subsystem2/1(In1)  "ADC_Acc_Z"
  Demux/4 -> Subsystem/1(In1)  "ADC_Temp"
  Demux/5 -> Subsystem4/1(In1)  "ADC_Gyro_X"
  Demux/6 -> Subsystem5/1(In1)  "ADC_Gyro_Y"
  Demux/7 -> Subsystem6/1(In1)  "ADC_Gyro_Z"
  Subsystem6/1(Out1) -> MPU6050_data_vector/7  "Gyro_Z [°/s]"
  Subsystem5/1(Out1) -> MPU6050_data_vector/6  "Gyro_Y [°/s]"
  Subsystem4/1(Out1) -> MPU6050_data_vector/5  "Gyro_X [°/s]"
  Subsystem/1(Out1) -> MPU6050_data_vector/4  "Temp [°C]"
  Subsystem2/1(Out1) -> MPU6050_data_vector/3  "Acc_Z [m/s^2]"
  Subsystem1/1(Out1) -> MPU6050_data_vector/2  "Acc_Y [m/s^2]"
  Subsystem3/1(Out1) -> MPU6050_data_vector/1  "Acc_X [m/s^2]"
  MPU6050_data_vector/1 -> MPU_data_vector/1  "MPU6050_data_vector"

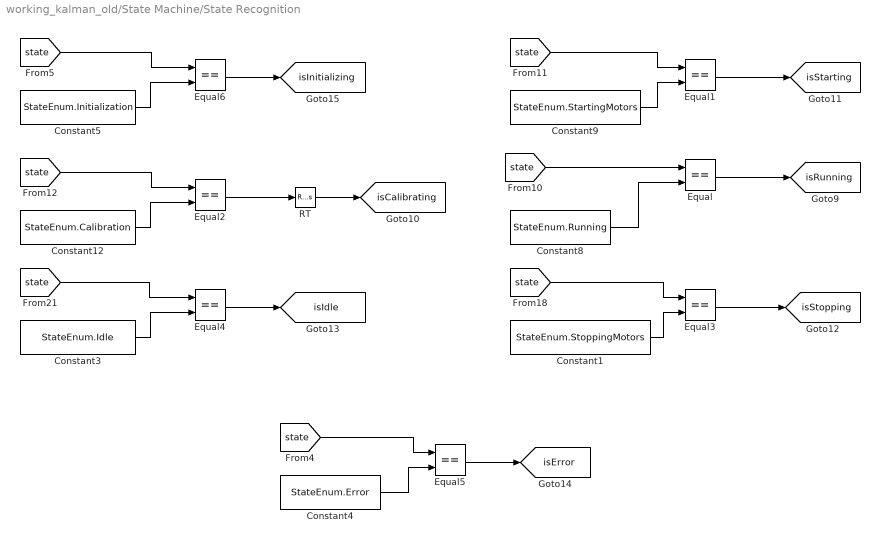
== system working_kalman_old/State Machine/State Recognition ==
  Constant1 : Constant  Value=StateEnum.StoppingMotors
  Constant12 : Constant  Value=StateEnum.Calibration
  Constant3 : Constant  Value=StateEnum.Idle
  Constant4 : Constant  Value=StateEnum.Error
  Constant5 : Constant  Value=StateEnum.Initialization
  Constant8 : Constant  Value=StateEnum.Running
  Constant9 : Constant  Value=StateEnum.StartingMotors
  Equal{,1..6} (7 alike) : RelationalOperator  Operator===  OutDataTypeStr=boolean  RndMeth=Simplest  InputSameDT=off
  RT : RateTransition  OutPortSampleTime=sensor_Ts
  tag scope: isCalibrating=global, isError=global, isIdle=global, isInitializing=global, isRunning=global, isStarting=global, isStopping=global
  wires:
  Equal2/1 -> RT/1
  [state] -> Equal4/1
  Equal6/1 -> [isInitializing]
  [state] -> Equal1/1
  Constant9/1 -> Equal1/2
  Constant12/1 -> Equal2/2
  Constant4/1 -> Equal5/2
  Constant8/1 -> Equal/2
  [state] -> Equal/1
  Equal4/1 -> [isIdle]
  Constant3/1 -> Equal4/2
  Constant5/1 -> Equal6/2
  Equal1/1 -> [isStarting]
  Equal/1 -> [isRunning]
  Constant1/1 -> Equal3/2
  [state] -> Equal2/1
  [state] -> Equal3/1
  Equal5/1 -> [isError]
  Equal3/1 -> [isStopping]
  [state] -> Equal6/1
  [state] -> Equal5/1
  RT/1 -> [isCalibrating]

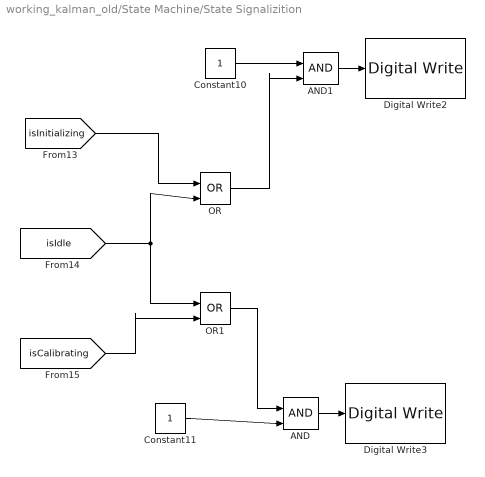
== system working_kalman_old/State Machine/State Signalizition ==
  AND : Logic  IconShape=distinctive  AllPortsSameDT=off  OutDataTypeStr=boolean
  AND1 : Logic  IconShape=distinctive  AllPortsSameDT=off  OutDataTypeStr=boolean
  Constant10 : Constant  OutDataTypeStr=boolean
  Constant11 : Constant  OutDataTypeStr=boolean
  Digital Write2 : mbedblockslib/Digital Write  Pin=LED3  Direction=output
      settings: LibrarySourceBlock=stmnucleorootlib/Common/Digital Write
  Digital Write3 : mbedblockslib/Digital Write  Pin=LED2  Direction=output
      settings: LibrarySourceBlock=stmnucleorootlib/Common/Digital Write
  OR : Logic  Operator=OR  IconShape=distinctive  AllPortsSameDT=off  OutDataTypeStr=boolean
  OR1 : Logic  Operator=OR  IconShape=distinctive  AllPortsSameDT=off  OutDataTypeStr=boolean
  wires:
  AND/1 -> Digital Write3/1
  [isInitializing] -> OR/1
  AND1/1 -> Digital Write2/1
  [isCalibrating] -> OR1/2
  [isIdle] -> OR1/1, OR/2
  Constant11/1 -> AND/2
  OR1/1 -> AND/1
  Constant10/1 -> AND1/1
  OR/1 -> AND1/2

== system working_kalman_old/State Machine/State Updates ==
  Detect Rise Positive : simulink/Logic and Bit Operations/Detect Rise Positive  vinit=0  OutDataTypeStr=boolean
  Digital Read : mbedblockslib/Digital Read  Pin=PC_13  Direction=input  SampleTime=simulink_Ts
      settings: LibrarySourceBlock=stmnucleorootlib/Common/Digital Read
  Equal : RelationalOperator  Operator===  OutDataTypeStr=boolean  RndMeth=Simplest  InputSameDT=off
  MATLAB Function2 : MATLAB Function  TreatAsAtomicUnit=on
  Seconds Counter : simulink/Sources/Counter Free-Running  NumBits=16  tsamp=1
  Unit Delay : UnitDelay  InitialCondition=stateInit  SampleTime=-1  HasFrameUpgradeWarning=on
  Unit Delay1 : UnitDelay  InitialCondition=init_time  SampleTime=-1  HasFrameUpgradeWarning=on
  tag scope: state=global
  wires:
  Unit Delay/1 -> [state]  "next_state"
  Digital Read/1 -> Detect Rise Positive/1
  [state] -> MATLAB Function2/1("state ")  "prev_state"
  Detect Rise Positive/1 -> MATLAB Function2/2(button_pushed)
  Seconds Counter/1 -> Equal/1, MATLAB Function2/3(seconds_counter)
  Equal/1 -> MATLAB Function2/4(time_elapsed)
  MATLAB Function2/2(time_when_elapsed) -> Unit Delay1/1
  Unit Delay1/1 -> MATLAB Function2/5("time_when_elapsed "), Equal/2
  MATLAB Function2/1(state) -> Unit Delay/1  "next_state"

== system working_kalman_old/Subsystem/Friction2 ==
  rad/s : Inport
  Gain : Gain  Gain=300
  Gain1 : Gain  Gain=friction_offset
  Gain2 : Gain  Gain=friction_slope
  Gain4 : Gain  Gain=1/(2*pi*60)
  Sum : Sum  Inputs=|++
  Tanh : Trigonometry  Operator=tanh
  friction : Outport
  wires:
  rad/s/1 -> Gain4/1
  Gain4/1 -> Gain2/1, Gain/1  "rpm"
  Gain1/1 -> Sum/1
  Tanh/1 -> Gain1/1
  Gain2/1 -> Sum/2
  Gain/1 -> Tanh/1
  Sum/1 -> friction/1

== system working_kalman_old/Subsystem/Friction3 ==
  rad/s : Inport
  Gain : Gain  Gain=300
  Gain1 : Gain  Gain=friction_offset
  Gain2 : Gain  Gain=friction_slope
  Gain4 : Gain  Gain=1/(2*pi*60)
  Sum : Sum  Inputs=|++
  Tanh : Trigonometry  Operator=tanh
  friction : Outport
  wires:
  rad/s/1 -> Gain4/1
  Gain4/1 -> Gain2/1, Gain/1  "rpm"
  Gain1/1 -> Sum/1
  Tanh/1 -> Gain1/1
  Gain2/1 -> Sum/2
  Gain/1 -> Tanh/1
  Sum/1 -> friction/1

== system working_kalman_old/CAN communication with B-G431-ESC1/Receive CAN Messages/Subsystem3 ==
  In1 : Inport
  Enable : EnablePort
  Byte Unpack : nucleoutilitieslib/Byte Unpack  dimensions={[2]}  datatypes={'single'}  byteAlign=1  blockPlatform=nucleo
  Out1 : Outport
  wires:
  Byte Unpack/1 -> Out1/1
  In1/1 -> Byte Unpack/1

== system working_kalman_old/CAN communication with B-G431-ESC1/Send CAN Messages/CAN_send ==
  data : Inport
  ID : Inport  Port=2
  Trigger : TriggerPort  VariantControl=(inherit)  PortDimensions=1
  CAN Pack : canmsglib/CAN Pack  MsgList=(none)  MsgName=LED_set  MsgIDType=Standard (11-bit identifier)  MsgIdentifier=hex2dec('7F3')  CANIDInput=on  MsgLength=8  Remote=off  ApplyMinMax=off  BusOutput=on  SignalInfo={}
      settings: LibrarySourceBlock=nucleoutilitieslib/CAN Pack  DataFormat=raw data
  CAN Transmit : stmnucleof7lib/CAN Transmit  CANModule=1  IdentifierType=Standard (11-bit identifier)  MsgId=hex2dec('7F3')  MsgLen=8  OutputStatus=on  RemoteFrame=off
      settings: DataFormat=CAN Message
  wires:
  CAN Pack/1 -> CAN Transmit/1
  data/1 -> CAN Pack/1
  ID/1 -> CAN Pack/2

== system working_kalman_old/CAN communication with B-G431-ESC1/Send CAN Messages/CAN_send1 ==
  data : Inport
  ID : Inport  Port=2
  Trigger : TriggerPort  VariantControl=(inherit)  PortDimensions=1
  CAN Pack : canmsglib/CAN Pack  MsgList=(none)  MsgName=LED_set  MsgIDType=Standard (11-bit identifier)  MsgIdentifier=hex2dec('7F3')  CANIDInput=on  MsgLength=8  Remote=off  ApplyMinMax=off  BusOutput=on  SignalInfo={}
      settings: LibrarySourceBlock=nucleoutilitieslib/CAN Pack  DataFormat=raw data
  CAN Transmit : stmnucleof7lib/CAN Transmit  CANModule=1  IdentifierType=Standard (11-bit identifier)  MsgId=hex2dec('7F3')  MsgLen=8  OutputStatus=on  RemoteFrame=off
      settings: DataFormat=CAN Message
  wires:
  CAN Pack/1 -> CAN Transmit/1
  data/1 -> CAN Pack/1
  ID/1 -> CAN Pack/2

== system working_kalman_old/CAN communication with B-G431-ESC1/Send CAN Messages/CAN_send2 ==
  data : Inport
  ID : Inport  Port=2
  Trigger : TriggerPort  VariantControl=(inherit)  PortDimensions=1
  CAN Pack : canmsglib/CAN Pack  MsgList=(none)  MsgName=LED_set  MsgIDType=Standard (11-bit identifier)  MsgIdentifier=hex2dec('7F3')  CANIDInput=on  MsgLength=8  Remote=off  ApplyMinMax=off  BusOutput=on  SignalInfo={}
      settings: LibrarySourceBlock=nucleoutilitieslib/CAN Pack  DataFormat=raw data
  CAN Transmit : stmnucleof7lib/CAN Transmit  CANModule=1  IdentifierType=Standard (11-bit identifier)  MsgId=hex2dec('7F3')  MsgLen=8  OutputStatus=on  RemoteFrame=off
      settings: DataFormat=CAN Message
  wires:
  CAN Pack/1 -> CAN Transmit/1
  data/1 -> CAN Pack/1
  ID/1 -> CAN Pack/2

== system working_kalman_old/CAN communication with B-G431-ESC1/Send CAN Messages/CAN_send3 ==
  data : Inport
  ID : Inport  Port=2
  Trigger : TriggerPort  VariantControl=(inherit)  PortDimensions=1
  CAN Pack : canmsglib/CAN Pack  MsgList=(none)  MsgName=LED_set  MsgIDType=Standard (11-bit identifier)  MsgIdentifier=hex2dec('7F3')  CANIDInput=on  MsgLength=8  Remote=off  ApplyMinMax=off  BusOutput=on  SignalInfo={}
      settings: LibrarySourceBlock=nucleoutilitieslib/CAN Pack  DataFormat=raw data
  CAN Transmit : stmnucleof7lib/CAN Transmit  CANModule=1  IdentifierType=Standard (11-bit identifier)  MsgId=hex2dec('7F3')  MsgLen=8  OutputStatus=on  RemoteFrame=off
      settings: DataFormat=CAN Message
  wires:
  CAN Pack/1 -> CAN Transmit/1
  data/1 -> CAN Pack/1
  ID/1 -> CAN Pack/2

== system working_kalman_old/CAN communication with B-G431-ESC1/Send CAN Messages/Set_speed1 ==
  Cast To Double : DataTypeConversion  OutDataTypeStr=uint8  SaturateOnIntegerOverflow=off  RndMeth=Floor
  Constant : Constant  Value=zeros(1,7)
  Constant5 : Constant  Value=hex2dec('7F3')
  Pulse Generator1 : DiscretePulseGenerator  PulseType=Time based  Period=1  PulseWidth=50
  Vector Concatenate : Concatenate
  data : Outport
  ID : Outport  Port=2
  wires:
  Constant5/1 -> ID/1
  Pulse Generator1/1 -> Vector Concatenate/1
  Vector Concatenate/1 -> Cast To Double/1
  Constant/1 -> Vector Concatenate/2
  Cast To Double/1 -> data/1

== system working_kalman_old/CAN communication with B-G431-ESC1/Send CAN Messages/Set_torque ==
  Byte Pack1 : nucleoutilitieslib/Byte Pack  datatypes={'uint16'}  byteAlign=1  blockPlatform=nucleo
  Byte Pack2 : nucleoutilitieslib/Byte Pack  datatypes={'single'}  byteAlign=1  blockPlatform=nucleo
  Cast : DataTypeConversion  OutDataTypeStr=single  SaturateOnIntegerOverflow=off  RndMeth=Floor
  Constant1 : Constant  Value=[0,0]  OutDataTypeStr=uint8  SampleTime=-1
  Constant5 : Constant  Value=hex2dec('043')
  Vector Concatenate3 : Concatenate  NumInputs=3
  final_speed [rpm] : Constant  Commented=on  Value=1200  OutDataTypeStr=single
  time_ramp [ms] : Constant  Value=0  OutDataTypeStr=uint16  SampleTime=-1
  data : Outport
  ID : Outport  Port=2
  wires:
  time_ramp [ms]/1 -> Byte Pack1/1
  Constant1/1 -> Vector Concatenate3/3
  Byte Pack1/1 -> Vector Concatenate3/2
  Byte Pack2/1 -> Vector Concatenate3/1
  Constant5/1 -> ID/1
  Vector Concatenate3/1 -> data/1
  [ramp_torque] -> Cast/1  "reference_torque [A]"
  Cast/1 -> Byte Pack2/1

== system working_kalman_old/CAN communication with B-G431-ESC1/Send CAN Messages/Start_Motor ==
  Constant3 : Constant  Value=[1,0,0,0,0,0,0,0]  OutDataTypeStr=uint8  SampleTime=-1
  Constant4 : Constant  Value=hex2dec('033')
  data : Outport
  ID : Outport  Port=2
  wires:
  Constant3/1 -> data/1
  Constant4/1 -> ID/1

== system working_kalman_old/CAN communication with B-G431-ESC1/Send CAN Messages/Stop_Motor ==
  Byte Pack1 : nucleoutilitieslib/Byte Pack  datatypes={'uint16'}  byteAlign=1  blockPlatform=nucleo
  Byte Pack2 : nucleoutilitieslib/Byte Pack  datatypes={'single'}  byteAlign=1  blockPlatform=nucleo
  Constant1 : Constant  Value=[0,0]  OutDataTypeStr=uint8  SampleTime=-1
  Constant3 : Constant  Value=[0,0,0,0,0,0,0,0]  OutDataTypeStr=uint8  SampleTime=-1
  Constant4 : Constant  Value=hex2dec('033')
  Constant5 : Constant  Value=hex2dec('023')
  Vector Concatenate3 : Concatenate  NumInputs=3
  final_speed [rpm] : Constant  Value=-1200  OutDataTypeStr=single
  time_ramp [ms] : Constant  OutDataTypeStr=uint16
  data : Outport
  ID : Outport  Port=2
  wires:
  Byte Pack2/1 -> Vector Concatenate3/1
  final_speed [rpm]/1 -> Byte Pack2/1
  time_ramp [ms]/1 -> Byte Pack1/1
  Byte Pack1/1 -> Vector Concatenate3/2
  Constant1/1 -> Vector Concatenate3/3
  Constant4/1 -> ID/1
  Constant3/1 -> data/1

== system working_kalman_old/ICM20948/Read sensing data/Subsystem ==
  In1 : Inport
  Add Constant : Bias  Bias=36.53  SaturateOnIntegerOverflow=off
  Cast To Double : DataTypeConversion  OutDataTypeStr=double  SaturateOnIntegerOverflow=off  RndMeth=Floor
  Gain7 : Gain  Gain=1/340
  Out1 : Outport
  wires:
  Gain7/1 -> Add Constant/1  "Temp"
  Add Constant/1 -> Out1/1
  In1/1 -> Cast To Double/1
  Cast To Double/1 -> Gain7/1

== system working_kalman_old/ICM20948/Read sensing data/Subsystem1 ==
  In1 : Inport
  8g range : Gain  Gain=9.81275/4096
  Cast To Double : DataTypeConversion  OutDataTypeStr=double  SaturateOnIntegerOverflow=off  RndMeth=Floor
  Offset : Bias  SaturateOnIntegerOverflow=off
  Out1 : Outport
  wires:
  Cast To Double/1 -> 8g range/1
  Offset/1 -> Out1/1
  In1/1 -> Cast To Double/1
  8g range/1 -> Offset/1  "Acc_Z"

== system working_kalman_old/ICM20948/Read sensing data/Subsystem2 ==
  In1 : Inport
  8g range : Gain  Gain=9.81275/4096
  Cast To Double : DataTypeConversion  OutDataTypeStr=double  SaturateOnIntegerOverflow=off  RndMeth=Floor
  Offset : Bias  SaturateOnIntegerOverflow=off
  Out1 : Outport
  wires:
  8g range/1 -> Offset/1  "Acc_Z"
  In1/1 -> Cast To Double/1
  Offset/1 -> Out1/1
  Cast To Double/1 -> 8g range/1

== system working_kalman_old/ICM20948/Read sensing data/Subsystem3 ==
  In1 : Inport
  8g range : Gain  Gain=9.81275/4096
  Cast To Double : DataTypeConversion  OutDataTypeStr=double  SaturateOnIntegerOverflow=off  RndMeth=Floor
  Offset : Bias  SaturateOnIntegerOverflow=off
  Out1 : Outport
  wires:
  8g range/1 -> Offset/1  "Acc_Z"
  In1/1 -> Cast To Double/1
  Offset/1 -> Out1/1
  Cast To Double/1 -> 8g range/1

== system working_kalman_old/ICM20948/Read sensing data/Subsystem4 ==
  In1 : Inport
  +-500 °/s range : Gain  Gain=1/65.5
  Cast To Double : DataTypeConversion  OutDataTypeStr=double  SaturateOnIntegerOverflow=off  RndMeth=Floor
  Offset : Bias  SaturateOnIntegerOverflow=off
  Out1 : Outport
  wires:
  Offset/1 -> Out1/1
  +-500 °/s range/1 -> Offset/1  "Acc_Z"
  Cast To Double/1 -> +-500 °/s range/1
  In1/1 -> Cast To Double/1

== system working_kalman_old/ICM20948/Read sensing data/Subsystem5 ==
  In1 : Inport
  +-500 °/s range : Gain  Gain=1/65.5
  Cast To Double : DataTypeConversion  OutDataTypeStr=double  SaturateOnIntegerOverflow=off  RndMeth=Floor
  Offset : Bias  SaturateOnIntegerOverflow=off
  Out1 : Outport
  wires:
  Offset/1 -> Out1/1
  +-500 °/s range/1 -> Offset/1  "Acc_Z"
  Cast To Double/1 -> +-500 °/s range/1
  In1/1 -> Cast To Double/1

== system working_kalman_old/ICM20948/Read sensing data/Subsystem6 ==
  In1 : Inport
  +-500 °/s range : Gain  Gain=1/65.5
  Cast To Double : DataTypeConversion  OutDataTypeStr=double  SaturateOnIntegerOverflow=off  RndMeth=Floor
  Offset : Bias  SaturateOnIntegerOverflow=off
  Out1 : Outport
  wires:
  Offset/1 -> Out1/1
  +-500 °/s range/1 -> Offset/1  "Acc_Z"
  Cast To Double/1 -> +-500 °/s range/1
  In1/1 -> Cast To Double/1

== system working_kalman_old/ICM42688-P/Measurement/Subsystem ==
  In1 : Inport
  Add Constant : Bias  Bias=25  SaturateOnIntegerOverflow=off
  Cast To Double : DataTypeConversion  OutDataTypeStr=double  SaturateOnIntegerOverflow=off  RndMeth=Floor
  Gain7 : Gain  Gain=1/132.48
  Out1 : Outport
  wires:
  Gain7/1 -> Add Constant/1  "Temp"
  Add Constant/1 -> Out1/1
  In1/1 -> Cast To Double/1
  Cast To Double/1 -> Gain7/1

== system working_kalman_old/ICM42688-P/Measurement/Subsystem1 ==
  In1 : Inport
  8g range : Gain  Gain=9.81275*16/(2^16-1)
  Cast To Double : DataTypeConversion  OutDataTypeStr=double  SaturateOnIntegerOverflow=off  RndMeth=Floor
  Offset : Bias  SaturateOnIntegerOverflow=off
  Out1 : Outport
  wires:
  Cast To Double/1 -> 8g range/1
  Offset/1 -> Out1/1
  In1/1 -> Cast To Double/1
  8g range/1 -> Offset/1  "Acc_X"

== system working_kalman_old/ICM42688-P/Measurement/Subsystem2 ==
  In1 : Inport
  8g range : Gain  Gain=9.81275*16/(2^16-1)
  Cast To Double : DataTypeConversion  OutDataTypeStr=double  SaturateOnIntegerOverflow=off  RndMeth=Floor
  Offset : Bias  SaturateOnIntegerOverflow=off
  Out1 : Outport
  wires:
  8g range/1 -> Offset/1  "Acc_Y"
  In1/1 -> Cast To Double/1
  Offset/1 -> Out1/1
  Cast To Double/1 -> 8g range/1

== system working_kalman_old/ICM42688-P/Measurement/Subsystem3 ==
  In1 : Inport
  8g range : Gain  Gain=9.81275*16/(2^16-1)
  Cast To Double : DataTypeConversion  OutDataTypeStr=double  SaturateOnIntegerOverflow=off  RndMeth=Floor
  Offset : Bias  SaturateOnIntegerOverflow=off
  Out1 : Outport
  wires:
  8g range/1 -> Offset/1  "Acc_Z"
  In1/1 -> Cast To Double/1
  Offset/1 -> Out1/1
  Cast To Double/1 -> 8g range/1

== system working_kalman_old/ICM42688-P/Measurement/Subsystem4 ==
  In1 : Inport
  +-1000 °/s range : Gain  Gain=2000/(2^16-1)
  Cast To Double : DataTypeConversion  OutDataTypeStr=double  SaturateOnIntegerOverflow=off  RndMeth=Floor
  Offset : Bias  SaturateOnIntegerOverflow=off
  Out1 : Outport
  wires:
  Offset/1 -> Out1/1
  +-1000 °/s range/1 -> Offset/1  "Gyr_X"
  Cast To Double/1 -> +-1000 °/s range/1
  In1/1 -> Cast To Double/1

== system working_kalman_old/ICM42688-P/Measurement/Subsystem5 ==
  In1 : Inport
  +-1000 °/s range1 : Gain  Gain=2000/(2^16-1)
  Cast To Double : DataTypeConversion  OutDataTypeStr=double  SaturateOnIntegerOverflow=off  RndMeth=Floor
  Offset : Bias  SaturateOnIntegerOverflow=off
  Out1 : Outport
  wires:
  Offset/1 -> Out1/1
  +-1000 °/s range1/1 -> Offset/1  "Gyr_Y"
  Cast To Double/1 -> +-1000 °/s range1/1
  In1/1 -> Cast To Double/1

== system working_kalman_old/ICM42688-P/Measurement/Subsystem6 ==
  In1 : Inport
  +-1000 °/s range : Gain  Gain=2000/(2^16-1)
  Cast To Double : DataTypeConversion  OutDataTypeStr=double  SaturateOnIntegerOverflow=off  RndMeth=Floor
  Offset : Bias  SaturateOnIntegerOverflow=off
  Out1 : Outport
  wires:
  Offset/1 -> Out1/1
  +-1000 °/s range/1 -> Offset/1  "Gyr_Z"
  Cast To Double/1 -> +-1000 °/s range/1
  In1/1 -> Cast To Double/1

== system working_kalman_old/MPU6050/Read sensing data/Subsystem ==
  In1 : Inport
  Add Constant : Bias  Bias=36.53  SaturateOnIntegerOverflow=off
  Cast To Double : DataTypeConversion  OutDataTypeStr=double  SaturateOnIntegerOverflow=off  RndMeth=Floor
  Gain7 : Gain  Gain=1/340
  Out1 : Outport
  wires:
  Gain7/1 -> Add Constant/1  "Temp"
  Add Constant/1 -> Out1/1
  In1/1 -> Cast To Double/1
  Cast To Double/1 -> Gain7/1

== system working_kalman_old/MPU6050/Read sensing data/Subsystem1 ==
  In1 : Inport
  8g range : Gain  Gain=9.81275/4096
  Cast To Double : DataTypeConversion  OutDataTypeStr=double  SaturateOnIntegerOverflow=off  RndMeth=Floor
  Offset : Bias  SaturateOnIntegerOverflow=off
  Out1 : Outport
  wires:
  Cast To Double/1 -> 8g range/1
  Offset/1 -> Out1/1
  In1/1 -> Cast To Double/1
  8g range/1 -> Offset/1  "Acc_Z"
